simulink library "aircraft_lib"  (Simulink 9.1)
settings: Solver=VariableStepAuto  StartTime=0.0  StopTime=10.0  RelTol=1e-3
undefined symbols (not defined in the file or in its folder): runway_alt
libraries: acparams_lib x2, actuator_lib x2, aero_lib x2, auxvars_lib x2, avionics_lib x2, eomlib x2, enginelib x2, gravity_lib x2, landinggear_lib x2, sensors_lib x2, $bdroot x1, simulink x1
settings Model: Creator=Austin Murch  LastModifiedBy=E183308  ExtModeAutoUpdateStatusClock=off

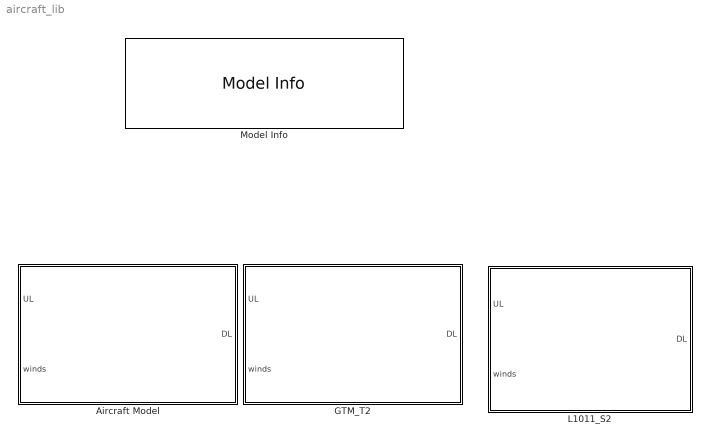
== system aircraft_lib ==
  Aircraft Model : Subsystem  BlockChoice=GTM_T2
      settings: TemplateBlock=self  MemberBlocks=GTM_T2,L1011_S2
  GTM_T2 : Subsystem  Tag=From trunk/GTMsim/gtm_model.mdl revision 162
      mask Display: image(imread('GTMtiny.png'))
  L1011_S2 : Subsystem  Tag=From trunk/GTMsim/gtm_model.mdl revision 162
      mask Display: image(imread('S2tiny.jpg'))
  Model Info : simulink/Model-Wide Utilities/Model Info  Frame=on  DisplayStringWithTags=|  HorizontalTextAlignment=Center  LeftAlignmentValue=0.5
      | Aircraft Plant Library
      | %<ModelVersion>
      | Las modified by %<LastModifiedBy> on %<LastModificationDate>

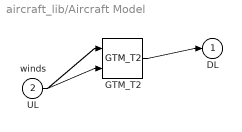
== system aircraft_lib/Aircraft Model ==
  UL : Inport
  winds : Inport  Port=2
  GTM_T2 : $bdroot/GTM_T2  Tag=From trunk/GTMsim/gtm_model.mdl revision 162  SystemSampleTime=-1
  DL : Outport
  wires:
  UL/1 -> GTM_T2/1
  winds/1 -> GTM_T2/2
  GTM_T2/1 -> DL/1

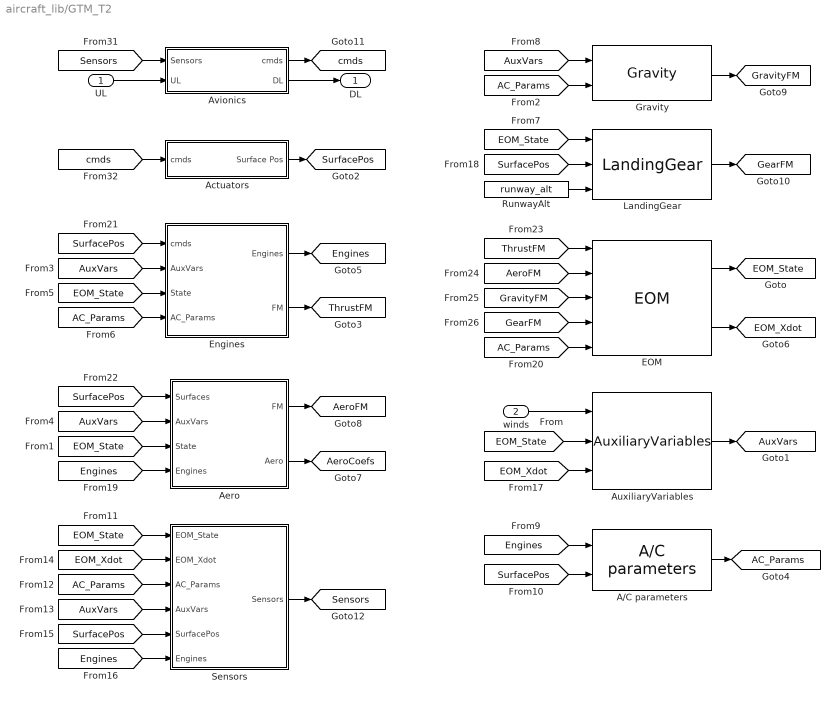
== system aircraft_lib/GTM_T2 ==
  UL : Inport
  winds : Inport  Port=2  PortDimensions=3
  A/C parameters : acparams_lib/A//C parameters  SystemSampleTime=-1
  Actuators : Subsystem  BlockChoice=GTM_T2
      settings: AttributesFormatString=%<BlockChoice>  TemplateBlock=actuator_lib/Actuators  MemberBlocks=FASER,GTM_T2,L1011_S2
  Aero : Subsystem  BlockChoice=GTM_T2
      settings: AttributesFormatString=%<BlockChoice>  TemplateBlock=aero_lib/Aero  MemberBlocks=FASER,GTM_T2,L1011_S2
  AuxiliaryVariables : auxvars_lib/AuxiliaryVariables  SystemSampleTime=-1
  Avionics : Subsystem  BlockChoice=GTM_T2
      settings: AttributesFormatString=%<BlockChoice>  TemplateBlock=avionics_lib/Avionics  MemberBlocks=Blank,GTM_T2,L1011_S2
  EOM : eomlib/EOM  SystemSampleTime=-1
  Engines : Subsystem  BlockChoice=GTM_T2
      link override GTM_T2/Left_Engine: BlockChoice=Jetcat P70
      link override GTM_T2/Right_Engine: BlockChoice=Jetcat P70
      settings: AttributesFormatString=%<BlockChoice>  TemplateBlock=enginelib/Engines  MemberBlocks=GTM_T2,L1011_S2
  Gravity : gravity_lib/Gravity  SystemSampleTime=-1
  LandingGear : landinggear_lib/LandingGear  SystemSampleTime=-1  GEAR_SPRING=25*12  zeta=0.4  NoseWheelRate=0.15
  RunwayAlt : Constant  Value=runway_alt
  Sensors : Subsystem  BlockChoice=GTM_T2
      settings: AttributesFormatString=%<BlockChoice>  TemplateBlock=sensors_lib/Sensors  MemberBlocks=Blank,GTM_T2,L1011_S2
  DL : Outport
  tag scope: AC_Params=global, AeroCoefs=global, AeroFM=global, AuxVars=global, EOM_State=global, EOM_Xdot=global, Engines=global, GearFM=global, GravityFM=global, Sensors=global, SurfacePos=global, ThrustFM=global, cmds=global
  wires:
  UL/1 -> Avionics/2(UL)
  Avionics/2(DL) -> DL/1
  Gravity/1 -> [GravityFM]
  [AuxVars] -> Sensors/4(AuxVars)
  [EOM_Xdot] -> Sensors/2(EOM_Xdot)
  [Engines] -> Sensors/6(Engines)
  [SurfacePos] -> Sensors/5(SurfacePos)
  [AC_Params] -> Sensors/3(AC_Params)
  [EOM_State] -> Sensors/1(EOM_State)
  [AC_Params] -> EOM/5
  [GearFM] -> EOM/4
  [GravityFM] -> EOM/3
  [AeroFM] -> EOM/2
  [ThrustFM] -> EOM/1
  [EOM_State] -> AuxiliaryVariables/2
  Aero/2(Aero) -> [AeroCoefs]
  [SurfacePos] -> Aero/1(Surfaces)
  RunwayAlt/1 -> LandingGear/3
  [SurfacePos] -> Engines/1(cmds)
  EOM/2 -> [EOM_Xdot]
  [Engines] -> Aero/4(Engines)
  [EOM_Xdot] -> AuxiliaryVariables/3
  Engines/1(Engines) -> [Engines]
  [SurfacePos] -> A/C parameters/2
  [Engines] -> A/C parameters/1
  A/C parameters/1 -> [AC_Params]
  [AC_Params] -> Engines/4(AC_Params)
  [AuxVars] -> Engines/2(AuxVars)
  [EOM_State] -> Engines/3(State)
  [AuxVars] -> Gravity/1
  [AC_Params] -> Gravity/2
  EOM/1 -> [EOM_State]
  Engines/2(FM) -> [ThrustFM]
  Aero/1(FM) -> [AeroFM]
  [AuxVars] -> Aero/2(AuxVars)
  AuxiliaryVariables/1 -> [AuxVars]
  [EOM_State] -> Aero/3(State)
  [EOM_State] -> LandingGear/1
  [SurfacePos] -> LandingGear/2
  LandingGear/1 -> [GearFM]
  Actuators/1(Surface Pos) -> [SurfacePos]
  winds/1 -> AuxiliaryVariables/1
  Avionics/1(cmds) -> [cmds]
  [Sensors] -> Avionics/1(Sensors)
  [cmds] -> Actuators/1(cmds)
  Sensors/1(Sensors) -> [Sensors]

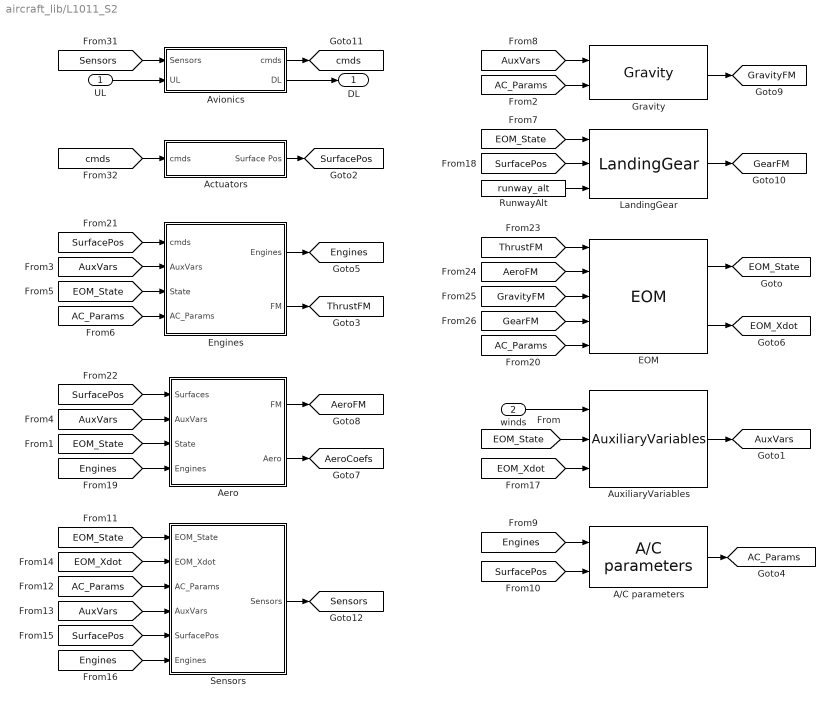
== system aircraft_lib/L1011_S2 ==
  UL : Inport
  winds : Inport  Port=2  PortDimensions=3
  A/C parameters : acparams_lib/A//C parameters  SystemSampleTime=-1
  Actuators : Subsystem  BlockChoice=L1011_S2
      settings: AttributesFormatString=%<BlockChoice>  TemplateBlock=actuator_lib/Actuators  MemberBlocks=FASER,GTM_T2,L1011_S2
  Aero : Subsystem  BlockChoice=L1011_S2
      settings: AttributesFormatString=%<BlockChoice>  TemplateBlock=aero_lib/Aero  MemberBlocks=FASER,GTM_T2,L1011_S2
  AuxiliaryVariables : auxvars_lib/AuxiliaryVariables  SystemSampleTime=-1
  Avionics : Subsystem  BlockChoice=L1011_S2
      settings: AttributesFormatString=%<BlockChoice>  TemplateBlock=avionics_lib/Avionics  MemberBlocks=Blank,GTM_T2,L1011_S2
  EOM : eomlib/EOM  SystemSampleTime=-1
  Engines : Subsystem  BlockChoice=L1011_S2
      settings: AttributesFormatString=%<BlockChoice>  TemplateBlock=enginelib/Engines  MemberBlocks=GTM_T2,L1011_S2
  Gravity : gravity_lib/Gravity  SystemSampleTime=-1
  LandingGear : landinggear_lib/LandingGear  SystemSampleTime=-1  GEAR_SPRING=25*12  zeta=0.4  NoseWheelRate=0.15
  RunwayAlt : Constant  Value=runway_alt
  Sensors : Subsystem  BlockChoice=L1011_S2
      settings: AttributesFormatString=%<BlockChoice>  TemplateBlock=sensors_lib/Sensors  MemberBlocks=Blank,GTM_T2,L1011_S2
  DL : Outport
  tag scope: AC_Params=global, AeroCoefs=global, AeroFM=global, AuxVars=global, EOM_State=global, EOM_Xdot=global, Engines=global, GearFM=global, GravityFM=global, Sensors=global, SurfacePos=global, ThrustFM=global, cmds=global
  wires:
  UL/1 -> Avionics/2(UL)
  Avionics/2(DL) -> DL/1
  Gravity/1 -> [GravityFM]
  [AuxVars] -> Sensors/4(AuxVars)
  [EOM_Xdot] -> Sensors/2(EOM_Xdot)
  [Engines] -> Sensors/6(Engines)
  [SurfacePos] -> Sensors/5(SurfacePos)
  [AC_Params] -> Sensors/3(AC_Params)
  [EOM_State] -> Sensors/1(EOM_State)
  [AC_Params] -> EOM/5
  [GearFM] -> EOM/4
  [GravityFM] -> EOM/3
  [AeroFM] -> EOM/2
  [ThrustFM] -> EOM/1
  [EOM_State] -> AuxiliaryVariables/2
  Aero/2(Aero) -> [AeroCoefs]
  [SurfacePos] -> Aero/1(Surfaces)
  RunwayAlt/1 -> LandingGear/3
  [SurfacePos] -> Engines/1(cmds)
  EOM/2 -> [EOM_Xdot]
  [Engines] -> Aero/4(Engines)
  [EOM_Xdot] -> AuxiliaryVariables/3
  Engines/1(Engines) -> [Engines]
  [SurfacePos] -> A/C parameters/2
  [Engines] -> A/C parameters/1
  A/C parameters/1 -> [AC_Params]
  [AC_Params] -> Engines/4(AC_Params)
  [AuxVars] -> Engines/2(AuxVars)
  [EOM_State] -> Engines/3(State)
  [AuxVars] -> Gravity/1
  [AC_Params] -> Gravity/2
  EOM/1 -> [EOM_State]
  Engines/2(FM) -> [ThrustFM]
  Aero/1(FM) -> [AeroFM]
  [AuxVars] -> Aero/2(AuxVars)
  AuxiliaryVariables/1 -> [AuxVars]
  [EOM_State] -> Aero/3(State)
  [EOM_State] -> LandingGear/1
  [SurfacePos] -> LandingGear/2
  LandingGear/1 -> [GearFM]
  Actuators/1(Surface Pos) -> [SurfacePos]
  winds/1 -> AuxiliaryVariables/1
  Avionics/1(cmds) -> [cmds]
  [Sensors] -> Avionics/1(Sensors)
  [cmds] -> Actuators/1(cmds)
  Sensors/1(Sensors) -> [Sensors]

== system aircraft_lib/GTM_T2/Actuators ==
  cmds : Inport
  GTM_T2 : actuator_lib/GTM_T2  SystemSampleTime=-1
  Surface Pos : Outport
  wires:
  GTM_T2/1 -> Surface Pos/1
  cmds/1 -> GTM_T2/1

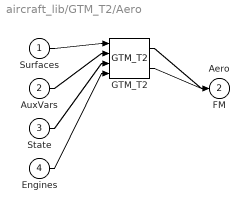
== system aircraft_lib/GTM_T2/Aero ==
  Surfaces : Inport
  AuxVars : Inport  Port=2
  State : Inport  Port=3
  Engines : Inport  Port=4
  GTM_T2 : aero_lib/GTM_T2  SystemSampleTime=-1
  FM : Outport
  Aero : Outport  Port=2
  wires:
  GTM_T2/2 -> Aero/1
  GTM_T2/1 -> FM/1
  Engines/1 -> GTM_T2/4
  State/1 -> GTM_T2/3
  AuxVars/1 -> GTM_T2/2
  Surfaces/1 -> GTM_T2/1

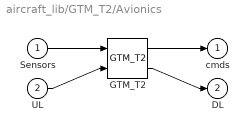
== system aircraft_lib/GTM_T2/Avionics ==
  Sensors : Inport
  UL : Inport  Port=2
  GTM_T2 : avionics_lib/GTM_T2  SystemSampleTime=-1
  cmds : Outport
  DL : Outport  Port=2
  wires:
  GTM_T2/2 -> DL/1
  GTM_T2/1 -> cmds/1
  UL/1 -> GTM_T2/2
  Sensors/1 -> GTM_T2/1

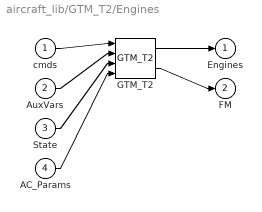
== system aircraft_lib/GTM_T2/Engines ==
  cmds : Inport
  AuxVars : Inport  Port=2
  State : Inport  Port=3
  AC_Params : Inport  Port=4
  GTM_T2 : enginelib/GTM_T2  SystemSampleTime=-1
  Engines : Outport
  FM : Outport  Port=2
  wires:
  cmds/1 -> GTM_T2/1
  AuxVars/1 -> GTM_T2/2
  State/1 -> GTM_T2/3
  AC_Params/1 -> GTM_T2/4
  GTM_T2/1 -> Engines/1
  GTM_T2/2 -> FM/1

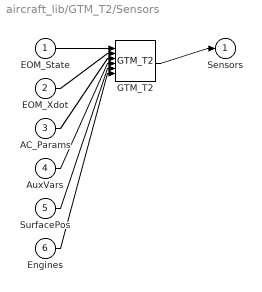
== system aircraft_lib/GTM_T2/Sensors ==
  EOM_State : Inport
  EOM_Xdot : Inport  Port=2
  AC_Params : Inport  Port=3
  AuxVars : Inport  Port=4
  SurfacePos : Inport  Port=5
  Engines : Inport  Port=6
  GTM_T2 : sensors_lib/GTM_T2  SystemSampleTime=-1
  Sensors : Outport
  wires:
  GTM_T2/1 -> Sensors/1
  Engines/1 -> GTM_T2/6
  SurfacePos/1 -> GTM_T2/5
  AuxVars/1 -> GTM_T2/4
  AC_Params/1 -> GTM_T2/3
  EOM_Xdot/1 -> GTM_T2/2
  EOM_State/1 -> GTM_T2/1

== system aircraft_lib/L1011_S2/Actuators ==
  cmds : Inport
  L1011_S2 : actuator_lib/L1011_S2  SystemSampleTime=-1
  Surface Pos : Outport
  wires:
  L1011_S2/1 -> Surface Pos/1
  cmds/1 -> L1011_S2/1

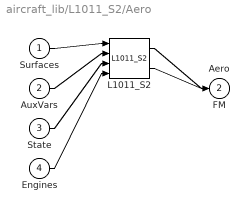
== system aircraft_lib/L1011_S2/Aero ==
  Surfaces : Inport
  AuxVars : Inport  Port=2
  State : Inport  Port=3
  Engines : Inport  Port=4
  L1011_S2 : aero_lib/L1011_S2  SystemSampleTime=-1
  FM : Outport
  Aero : Outport  Port=2
  wires:
  L1011_S2/2 -> Aero/1
  L1011_S2/1 -> FM/1
  Engines/1 -> L1011_S2/4
  State/1 -> L1011_S2/3
  AuxVars/1 -> L1011_S2/2
  Surfaces/1 -> L1011_S2/1

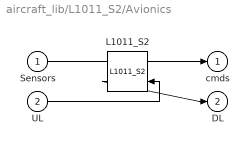
== system aircraft_lib/L1011_S2/Avionics ==
  Sensors : Inport
  UL : Inport  Port=2
  L1011_S2 : avionics_lib/L1011_S2  SystemSampleTime=-1
  cmds : Outport
  DL : Outport  Port=2
  wires:
  L1011_S2/2 -> DL/1
  L1011_S2/1 -> cmds/1
  UL/1 -> L1011_S2/2
  Sensors/1 -> L1011_S2/1

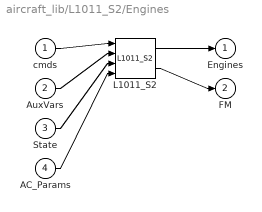
== system aircraft_lib/L1011_S2/Engines ==
  cmds : Inport
  AuxVars : Inport  Port=2
  State : Inport  Port=3
  AC_Params : Inport  Port=4
  L1011_S2 : enginelib/L1011_S2  SystemSampleTime=-1
  Engines : Outport
  FM : Outport  Port=2
  wires:
  L1011_S2/2 -> FM/1
  L1011_S2/1 -> Engines/1
  AC_Params/1 -> L1011_S2/4
  State/1 -> L1011_S2/3
  AuxVars/1 -> L1011_S2/2
  cmds/1 -> L1011_S2/1

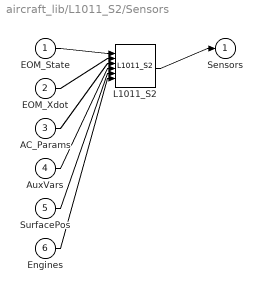
== system aircraft_lib/L1011_S2/Sensors ==
  EOM_State : Inport
  EOM_Xdot : Inport  Port=2
  AC_Params : Inport  Port=3
  AuxVars : Inport  Port=4
  SurfacePos : Inport  Port=5
  Engines : Inport  Port=6
  L1011_S2 : sensors_lib/L1011_S2  SystemSampleTime=-1
  Sensors : Outport
  wires:
  L1011_S2/1 -> Sensors/1
  Engines/1 -> L1011_S2/6
  SurfacePos/1 -> L1011_S2/5
  AuxVars/1 -> L1011_S2/4
  AC_Params/1 -> L1011_S2/3
  EOM_Xdot/1 -> L1011_S2/2
  EOM_State/1 -> L1011_S2/1
